simulink model "Katex_FullCar_R2017b_V03"  (R2026a)
settings: Solver=ode1  StopTime=1000  FixedStep=Ts  EnableMultiTasking=on
PostLoadFcn:
  | , if any(exist('dsrtsu_mdlpostloadfcn', 'file') == [2, 3, 6]), try dsrtsu_mdlpostloadfcn('Execute', bdroot); catch fprintf('Error in PostLoadFcn (dsrtsu_mdlpostloadfcn) for model "%s":\n %s\n', bdroot, lasterr); end, end,
  | , if any(exist('dsrtsu_mdlpostloadfcn', 'file') ~= 0), dsrtsu_mdlpostloadfcn('Execute', bdroot); end,
InitFcn:
  | , if any(exist('rtifpga_mdlclblib', 'file') ~= 0), rtifpga_mdlclblib('Init', bdroot); end,
  | 
  | 
  | init
undefined symbols (not defined in the file): locklim_sus, roundN, Ts
libraries: sl_discontinuities x29, simulink_extras x26, simulink x22, mjLib x1
(part 7 of 10)

== system Katex_FullCar_R2017b_V03/DGIST/_Low_Level_Ctrl/Suspension_Low_Level_Controller/Velocity Mode/Sus_LoadVel_2_MotorRPM/LPF2 ==
  note: LPF : tau = 1/(2*pi*fc)
  note: y(n) = [Ts*{x(n)+x(n-1)}+(2*tau-Ts)*y(n-1)]/(2*tau+Ts)
  note: H(s) = 1/(tau*s+1)
  note: s = 2/Ts*(z-1)/(z+1)
  In : Inport
  fc : Inport  Port=2
  Constant : Constant  Value=Ts  SampleTime=Ts
  Constant1 : Constant  SampleTime=Ts
  Product1 : Product  Inputs=*/  RndMeth=Zero
  Product11 : Product  RndMeth=Zero
  Product2 : Product  Inputs=*/  RndMeth=Zero
  Sum1 : Sum  Inputs=+-  InputSameDT=on  SaturateOnIntegerOverflow=on  OutDataTypeStr=Inherit: Same as first input
  Sum2 : Sum  InputSameDT=on  SaturateOnIntegerOverflow=on  OutDataTypeStr=Inherit: Same as first input
  Sum3 : Sum  InputSameDT=on  SaturateOnIntegerOverflow=on  OutDataTypeStr=Inherit: Same as first input
  Sum4 : Sum  InputSameDT=on  SaturateOnIntegerOverflow=on  OutDataTypeStr=Inherit: Same as first input
  d : UnitDelay  SampleTime=Ts
  d1 : UnitDelay  SampleTime=Ts
  gain : Gain  Gain=Ts  SaturateOnIntegerOverflow=on  OutDataTypeStr=Inherit: Same as input  ParamDataTypeStr=Inherit: Same as input
  gain1 : Gain  Gain=2  SaturateOnIntegerOverflow=on  OutDataTypeStr=Inherit: Same as input  ParamDataTypeStr=Inherit: Same as input
  gain2 : Gain  Gain=2*pi  SaturateOnIntegerOverflow=on  OutDataTypeStr=Inherit: Same as input  ParamDataTypeStr=Inherit: Same as input
  Out : Outport  VectorParamsAs1DForOutWhenUnconnected=off
  wires:
  In/1 -> Sum3/1, d1/1
  d1/1 -> Sum3/2
  Sum3/1 -> gain/1
  gain/1 -> Sum2/1
  Product11/1 -> Sum2/2
  Sum1/1 -> Product11/1
  Constant/1 -> Sum1/2, Sum4/2
  fc/1 -> gain2/1
  gain1/1 -> Sum1/1, Sum4/1
  d/1 -> Product11/2
  Sum2/1 -> Product1/1
  Sum4/1 -> Product1/2
  Product1/1 -> Out/1, d/1
  Product2/1 -> gain1/1
  Constant1/1 -> Product2/1
  gain2/1 -> Product2/2

== system Katex_FullCar_R2017b_V03/DGIST/_Low_Level_Ctrl/Suspension_Low_Level_Controller/Velocity Mode/Sus_LoadVel_2_MotorRPM1/LPF2 ==
  note: LPF : tau = 1/(2*pi*fc)
  note: y(n) = [Ts*{x(n)+x(n-1)}+(2*tau-Ts)*y(n-1)]/(2*tau+Ts)
  note: H(s) = 1/(tau*s+1)
  note: s = 2/Ts*(z-1)/(z+1)
  In : Inport
  fc : Inport  Port=2
  Constant : Constant  Value=Ts  SampleTime=Ts
  Constant1 : Constant  SampleTime=Ts
  Product1 : Product  Inputs=*/  RndMeth=Zero
  Product11 : Product  RndMeth=Zero
  Product2 : Product  Inputs=*/  RndMeth=Zero
  Sum1 : Sum  Inputs=+-  InputSameDT=on  SaturateOnIntegerOverflow=on  OutDataTypeStr=Inherit: Same as first input
  Sum2 : Sum  InputSameDT=on  SaturateOnIntegerOverflow=on  OutDataTypeStr=Inherit: Same as first input
  Sum3 : Sum  InputSameDT=on  SaturateOnIntegerOverflow=on  OutDataTypeStr=Inherit: Same as first input
  Sum4 : Sum  InputSameDT=on  SaturateOnIntegerOverflow=on  OutDataTypeStr=Inherit: Same as first input
  d : UnitDelay  SampleTime=Ts
  d1 : UnitDelay  SampleTime=Ts
  gain : Gain  Gain=Ts  SaturateOnIntegerOverflow=on  OutDataTypeStr=Inherit: Same as input  ParamDataTypeStr=Inherit: Same as input
  gain1 : Gain  Gain=2  SaturateOnIntegerOverflow=on  OutDataTypeStr=Inherit: Same as input  ParamDataTypeStr=Inherit: Same as input
  gain2 : Gain  Gain=2*pi  SaturateOnIntegerOverflow=on  OutDataTypeStr=Inherit: Same as input  ParamDataTypeStr=Inherit: Same as input
  Out : Outport  VectorParamsAs1DForOutWhenUnconnected=off
  wires:
  In/1 -> Sum3/1, d1/1
  d1/1 -> Sum3/2
  Sum3/1 -> gain/1
  gain/1 -> Sum2/1
  Product11/1 -> Sum2/2
  Sum1/1 -> Product11/1
  Constant/1 -> Sum1/2, Sum4/2
  fc/1 -> gain2/1
  gain1/1 -> Sum1/1, Sum4/1
  d/1 -> Product11/2
  Sum2/1 -> Product1/1
  Sum4/1 -> Product1/2
  Product1/1 -> Out/1, d/1
  Product2/1 -> gain1/1
  Constant1/1 -> Product2/1
  gain2/1 -> Product2/2

== system Katex_FullCar_R2017b_V03/DGIST/_Low_Level_Ctrl/Suspension_Low_Level_Controller/Velocity Mode/Sus_LoadVel_2_MotorRPM2/LPF2 ==
  note: LPF : tau = 1/(2*pi*fc)
  note: y(n) = [Ts*{x(n)+x(n-1)}+(2*tau-Ts)*y(n-1)]/(2*tau+Ts)
  note: H(s) = 1/(tau*s+1)
  note: s = 2/Ts*(z-1)/(z+1)
  In : Inport
  fc : Inport  Port=2
  Constant : Constant  Value=Ts  SampleTime=Ts
  Constant1 : Constant  SampleTime=Ts
  Product1 : Product  Inputs=*/  RndMeth=Zero
  Product11 : Product  RndMeth=Zero
  Product2 : Product  Inputs=*/  RndMeth=Zero
  Sum1 : Sum  Inputs=+-  InputSameDT=on  SaturateOnIntegerOverflow=on  OutDataTypeStr=Inherit: Same as first input
  Sum2 : Sum  InputSameDT=on  SaturateOnIntegerOverflow=on  OutDataTypeStr=Inherit: Same as first input
  Sum3 : Sum  InputSameDT=on  SaturateOnIntegerOverflow=on  OutDataTypeStr=Inherit: Same as first input
  Sum4 : Sum  InputSameDT=on  SaturateOnIntegerOverflow=on  OutDataTypeStr=Inherit: Same as first input
  d : UnitDelay  SampleTime=Ts
  d1 : UnitDelay  SampleTime=Ts
  gain : Gain  Gain=Ts  SaturateOnIntegerOverflow=on  OutDataTypeStr=Inherit: Same as input  ParamDataTypeStr=Inherit: Same as input
  gain1 : Gain  Gain=2  SaturateOnIntegerOverflow=on  OutDataTypeStr=Inherit: Same as input  ParamDataTypeStr=Inherit: Same as input
  gain2 : Gain  Gain=2*pi  SaturateOnIntegerOverflow=on  OutDataTypeStr=Inherit: Same as input  ParamDataTypeStr=Inherit: Same as input
  Out : Outport  VectorParamsAs1DForOutWhenUnconnected=off
  wires:
  In/1 -> Sum3/1, d1/1
  d1/1 -> Sum3/2
  Sum3/1 -> gain/1
  gain/1 -> Sum2/1
  Product11/1 -> Sum2/2
  Sum1/1 -> Product11/1
  Constant/1 -> Sum1/2, Sum4/2
  fc/1 -> gain2/1
  gain1/1 -> Sum1/1, Sum4/1
  d/1 -> Product11/2
  Sum2/1 -> Product1/1
  Sum4/1 -> Product1/2
  Product1/1 -> Out/1, d/1
  Product2/1 -> gain1/1
  Constant1/1 -> Product2/1
  gain2/1 -> Product2/2

== system Katex_FullCar_R2017b_V03/DGIST/_Low_Level_Ctrl/Suspension_Low_Level_Controller/Velocity Mode/Sus_LoadVel_2_MotorRPM3/LPF2 ==
  note: LPF : tau = 1/(2*pi*fc)
  note: y(n) = [Ts*{x(n)+x(n-1)}+(2*tau-Ts)*y(n-1)]/(2*tau+Ts)
  note: H(s) = 1/(tau*s+1)
  note: s = 2/Ts*(z-1)/(z+1)
  In : Inport
  fc : Inport  Port=2
  Constant : Constant  Value=Ts  SampleTime=Ts
  Constant1 : Constant  SampleTime=Ts
  Product1 : Product  Inputs=*/  RndMeth=Zero
  Product11 : Product  RndMeth=Zero
  Product2 : Product  Inputs=*/  RndMeth=Zero
  Sum1 : Sum  Inputs=+-  InputSameDT=on  SaturateOnIntegerOverflow=on  OutDataTypeStr=Inherit: Same as first input
  Sum2 : Sum  InputSameDT=on  SaturateOnIntegerOverflow=on  OutDataTypeStr=Inherit: Same as first input
  Sum3 : Sum  InputSameDT=on  SaturateOnIntegerOverflow=on  OutDataTypeStr=Inherit: Same as first input
  Sum4 : Sum  InputSameDT=on  SaturateOnIntegerOverflow=on  OutDataTypeStr=Inherit: Same as first input
  d : UnitDelay  SampleTime=Ts
  d1 : UnitDelay  SampleTime=Ts
  gain : Gain  Gain=Ts  SaturateOnIntegerOverflow=on  OutDataTypeStr=Inherit: Same as input  ParamDataTypeStr=Inherit: Same as input
  gain1 : Gain  Gain=2  SaturateOnIntegerOverflow=on  OutDataTypeStr=Inherit: Same as input  ParamDataTypeStr=Inherit: Same as input
  gain2 : Gain  Gain=2*pi  SaturateOnIntegerOverflow=on  OutDataTypeStr=Inherit: Same as input  ParamDataTypeStr=Inherit: Same as input
  Out : Outport  VectorParamsAs1DForOutWhenUnconnected=off
  wires:
  In/1 -> Sum3/1, d1/1
  d1/1 -> Sum3/2
  Sum3/1 -> gain/1
  gain/1 -> Sum2/1
  Product11/1 -> Sum2/2
  Sum1/1 -> Product11/1
  Constant/1 -> Sum1/2, Sum4/2
  fc/1 -> gain2/1
  gain1/1 -> Sum1/1, Sum4/1
  d/1 -> Product11/2
  Sum2/1 -> Product1/1
  Sum4/1 -> Product1/2
  Product1/1 -> Out/1, d/1
  Product2/1 -> gain1/1
  Constant1/1 -> Product2/1
  gain2/1 -> Product2/2

== system Katex_FullCar_R2017b_V03/MuJoCo Interface/FL_Motor_Control/Drv_Driver/Velocity Mode/FL_vel_velocity_motor_driver/poleplacement(PI)1 ==
  error : Inport
  zeta : Inport  Port=2
  freq : Inport  Port=3
  anti_windup : Inport  Port=4
  2*zeta*wn*J : Product  Inputs=3
  2*zeta*wn*J1 : Product
  2*zeta*wn*J2 : Product
  Add : Sum  Inputs=+-
  Add1 : Sum
  Constant3 : Constant  Value=0.05
  Constant4 : Constant  Value=0.9
  Display : Display
  Display1 : Display
  Gain : Gain  Gain=2
  Integ : Subsystem
  Product : Product  Inputs=*/
  Sum : Sum  Inputs=|+-
  Unit Delay : UnitDelay  SampleTime=-1
  wn : Gain  Gain=2*pi
  wn^2*J : Product  Inputs=3
  controlgain : Outport
  wires:
  Unit Delay/1 -> Sum/2
  [local_Kp] -> Product/2
  Product/1 -> Unit Delay/1
  anti_windup/1 -> Product/1
  Sum/1 -> Integ/1(error)
  2*zeta*wn*J1/1 -> Add1/2
  2*zeta*wn*J2/1 -> Add1/1
  Add1/1 -> controlgain/1
  [local_Kp] -> 2*zeta*wn*J2/1
  [local_Ki] -> 2*zeta*wn*J1/2
  Integ/1(Out1) -> 2*zeta*wn*J1/1
  error/1 -> 2*zeta*wn*J2/2, Sum/1
  wn^2*J/1 -> Display1/1, [local_Ki]
  [Local_J] -> wn^2*J/3
  Add/1 -> Display/1, [local_Kp]
  wn/1 -> wn^2*J/1, wn^2*J/2, 2*zeta*wn*J/3
  Gain/1 -> 2*zeta*wn*J/1
  zeta/1 -> Gain/1
  [Local_J] -> 2*zeta*wn*J/2
  2*zeta*wn*J/1 -> Add/1
  [Local_B] -> Add/2
  freq/1 -> wn/1
  Constant4/1 -> [Local_B]
  Constant3/1 -> [Local_J]

== system Katex_FullCar_R2017b_V03/MuJoCo Interface/FL_Motor_Control/Str_Driver/Position Mode/FL_str_position_motor_driver/poleplacement(PD)+I ==
  error : Inport
  zeta : Inport  Port=2
  freq : Inport  Port=3
  velocity_rad_s : Inport  Port=4
  2*zeta*wn*J : Product  Inputs=3
  2*zeta*wn*J1 : Product
  2*zeta*wn*J2 : Product
  Add : Sum  Inputs=+-
  Add1 : Sum
  Constant3 : Constant
  Constant4 : Constant  Value=10
  Display : Display
  Display1 : Display
  Gain : Gain  Gain=2
  Gain1 : Gain  Gain=-1
  Saturation5 : Saturate  UpperLimit=100  LowerLimit=-100
  wn : Gain  Gain=2*pi
  wn^2*J : Product  Inputs=3
  controlgain : Outport
  wires:
  2*zeta*wn*J1/1 -> Add1/2
  Saturation5/1 -> controlgain/1  "Usat"
  Add1/1 -> Saturation5/1
  Gain1/1 -> 2*zeta*wn*J1/2
  2*zeta*wn*J2/1 -> Add1/1
  [local_Kp] -> 2*zeta*wn*J2/1
  [local_Kd] -> Gain1/1
  error/1 -> 2*zeta*wn*J2/2
  wn^2*J/1 -> Display1/1, [local_Kp]
  [Local_J] -> wn^2*J/3
  Add/1 -> Display/1, [local_Kd]
  wn/1 -> wn^2*J/1, wn^2*J/2, 2*zeta*wn*J/3
  Gain/1 -> 2*zeta*wn*J/1
  zeta/1 -> Gain/1
  [Local_J] -> 2*zeta*wn*J/2
  2*zeta*wn*J/1 -> Add/1
  [Local_B] -> Add/2
  freq/1 -> wn/1
  Constant4/1 -> [Local_B]
  Constant3/1 -> [Local_J]
  velocity_rad_s/1 -> 2*zeta*wn*J1/1

== system Katex_FullCar_R2017b_V03/MuJoCo Interface/FL_Motor_Control/Sus_Driver/Position Mode/FL_sus_position_motor_driver/poleplacement(PD)+I ==
  error : Inport
  zeta : Inport  Port=2
  freq : Inport  Port=3
  velocity_rad_s : Inport  Port=4
  2*zeta*wn*J : Product  Inputs=3
  2*zeta*wn*J1 : Product
  2*zeta*wn*J2 : Product
  Add : Sum  Inputs=+-
  Add1 : Sum  Inputs=+++
  Add2 : Sum  Inputs=+-
  Constant : Constant
  Constant3 : Constant  Value=0.05
  Constant4 : Constant  Value=1.05
  Display : Display
  Display1 : Display
  Gain : Gain  Gain=2
  Gain1 : Gain  Gain=-1
  Integ : Subsystem
  Product : Product  Inputs=*/
  Saturation5 : Saturate  UpperLimit=100  LowerLimit=-100
  Sum : Sum  Inputs=|+-
  Unit Delay : UnitDelay  SampleTime=-1
  ki : Product
  wn : Gain  Gain=2*pi
  wn^2*J : Product  Inputs=3
  controlgain : Outport
  wires:
  Constant3/1 -> [Local_J]
  Constant4/1 -> [Local_B]
  freq/1 -> wn/1
  [Local_B] -> Add/2
  2*zeta*wn*J/1 -> Add/1
  [Local_J] -> 2*zeta*wn*J/2
  zeta/1 -> Gain/1
  Gain/1 -> 2*zeta*wn*J/1
  wn/1 -> 2*zeta*wn*J/3, wn^2*J/2, wn^2*J/1
  Add/1 -> [local_Kd], Display/1
  [Local_J] -> wn^2*J/3
  wn^2*J/1 -> [local_Kp], Display1/1
  error/1 -> 2*zeta*wn*J2/2, Sum/1
  [local_Kd] -> Gain1/1
  [local_Kp] -> 2*zeta*wn*J2/1
  2*zeta*wn*J2/1 -> Add1/1
  Gain1/1 -> 2*zeta*wn*J1/2
  2*zeta*wn*J1/1 -> Add1/3
  ki/1 -> Add1/2
  Constant/1 -> ki/2
  Integ/1(Out1) -> ki/1
  Add1/1 -> Add2/1, Saturation5/1
  Saturation5/1 -> Add2/2, controlgain/1  "Usat"
  Add2/1 -> Product/1
  [local_Kp] -> Product/2
  Sum/1 -> Integ/1(error)
  Product/1 -> Unit Delay/1
  Unit Delay/1 -> Sum/2
  velocity_rad_s/1 -> 2*zeta*wn*J1/1

== system Katex_FullCar_R2017b_V03/MuJoCo Interface/FR_Motor_Control/Drv_Driver/Velocity Mode/FR_vel_velocity_motor_driver/poleplacement(PI)1 ==
  error : Inport
  zeta : Inport  Port=2
  freq : Inport  Port=3
  anti_windup : Inport  Port=4
  2*zeta*wn*J : Product  Inputs=3
  2*zeta*wn*J1 : Product
  2*zeta*wn*J2 : Product
  Add : Sum  Inputs=+-
  Add1 : Sum
  Constant3 : Constant  Value=0.05
  Constant4 : Constant  Value=0.9
  Display : Display
  Display1 : Display
  Gain : Gain  Gain=2
  Integ : Subsystem
  Product : Product  Inputs=*/
  Sum : Sum  Inputs=|+-
  Unit Delay : UnitDelay  SampleTime=-1
  wn : Gain  Gain=2*pi
  wn^2*J : Product  Inputs=3
  controlgain : Outport
  wires:
  Constant3/1 -> [Local_J]
  Constant4/1 -> [Local_B]
  freq/1 -> wn/1
  [Local_B] -> Add/2
  2*zeta*wn*J/1 -> Add/1
  [Local_J] -> 2*zeta*wn*J/2
  zeta/1 -> Gain/1
  Gain/1 -> 2*zeta*wn*J/1
  wn/1 -> 2*zeta*wn*J/3, wn^2*J/2, wn^2*J/1
  Add/1 -> [local_Kp], Display/1
  [Local_J] -> wn^2*J/3
  wn^2*J/1 -> [local_Ki], Display1/1
  error/1 -> Sum/1, 2*zeta*wn*J2/2
  Integ/1(Out1) -> 2*zeta*wn*J1/1
  [local_Ki] -> 2*zeta*wn*J1/2
  [local_Kp] -> 2*zeta*wn*J2/1
  Add1/1 -> controlgain/1
  2*zeta*wn*J2/1 -> Add1/1
  2*zeta*wn*J1/1 -> Add1/2
  Sum/1 -> Integ/1(error)
  anti_windup/1 -> Product/1
  Product/1 -> Unit Delay/1
  [local_Kp] -> Product/2
  Unit Delay/1 -> Sum/2

== system Katex_FullCar_R2017b_V03/MuJoCo Interface/FR_Motor_Control/Str_Driver/Position Mode/FR_str_position_motor_driver/poleplacement(PD)+I ==
  error : Inport
  zeta : Inport  Port=2
  freq : Inport  Port=3
  velocity_rad_s : Inport  Port=4
  2*zeta*wn*J : Product  Inputs=3
  2*zeta*wn*J1 : Product
  2*zeta*wn*J2 : Product
  Add : Sum  Inputs=+-
  Add1 : Sum
  Constant3 : Constant
  Constant4 : Constant  Value=10
  Display : Display
  Display1 : Display
  Gain : Gain  Gain=2
  Gain1 : Gain  Gain=-1
  Saturation5 : Saturate  UpperLimit=100  LowerLimit=-100
  wn : Gain  Gain=2*pi
  wn^2*J : Product  Inputs=3
  controlgain : Outport
  wires:
  velocity_rad_s/1 -> 2*zeta*wn*J1/1
  Constant3/1 -> [Local_J]
  Constant4/1 -> [Local_B]
  freq/1 -> wn/1
  [Local_B] -> Add/2
  2*zeta*wn*J/1 -> Add/1
  [Local_J] -> 2*zeta*wn*J/2
  zeta/1 -> Gain/1
  Gain/1 -> 2*zeta*wn*J/1
  wn/1 -> 2*zeta*wn*J/3, wn^2*J/2, wn^2*J/1
  Add/1 -> [local_Kd], Display/1
  [Local_J] -> wn^2*J/3
  wn^2*J/1 -> [local_Kp], Display1/1
  error/1 -> 2*zeta*wn*J2/2
  [local_Kd] -> Gain1/1
  [local_Kp] -> 2*zeta*wn*J2/1
  2*zeta*wn*J2/1 -> Add1/1
  Gain1/1 -> 2*zeta*wn*J1/2
  Add1/1 -> Saturation5/1
  Saturation5/1 -> controlgain/1  "Usat"
  2*zeta*wn*J1/1 -> Add1/2

== system Katex_FullCar_R2017b_V03/MuJoCo Interface/FR_Motor_Control/Sus_Driver/Position Mode/FR_sus_position_motor_driver/poleplacement(PD)+I ==
  error : Inport
  zeta : Inport  Port=2
  freq : Inport  Port=3
  velocity_rad_s : Inport  Port=4
  2*zeta*wn*J : Product  Inputs=3
  2*zeta*wn*J1 : Product
  2*zeta*wn*J2 : Product
  Add : Sum  Inputs=+-
  Add1 : Sum  Inputs=+++
  Add2 : Sum  Inputs=+-
  Constant : Constant
  Constant3 : Constant  Value=0.05
  Constant4 : Constant  Value=1.05
  Display : Display
  Display1 : Display
  Gain : Gain  Gain=2
  Gain1 : Gain  Gain=-1
  Integ : Subsystem
  Product : Product  Inputs=*/
  Saturation5 : Saturate  UpperLimit=100  LowerLimit=-100
  Sum : Sum  Inputs=|+-
  Unit Delay : UnitDelay  SampleTime=-1
  ki : Product
  wn : Gain  Gain=2*pi
  wn^2*J : Product  Inputs=3
  controlgain : Outport
  wires:
  velocity_rad_s/1 -> 2*zeta*wn*J1/1
  Unit Delay/1 -> Sum/2
  Product/1 -> Unit Delay/1
  Sum/1 -> Integ/1(error)
  [local_Kp] -> Product/2
  Add2/1 -> Product/1
  Saturation5/1 -> controlgain/1, Add2/2  "Usat"
  Add1/1 -> Saturation5/1, Add2/1
  Integ/1(Out1) -> ki/1
  Constant/1 -> ki/2
  ki/1 -> Add1/2
  2*zeta*wn*J1/1 -> Add1/3
  Gain1/1 -> 2*zeta*wn*J1/2
  2*zeta*wn*J2/1 -> Add1/1
  [local_Kp] -> 2*zeta*wn*J2/1
  [local_Kd] -> Gain1/1
  error/1 -> Sum/1, 2*zeta*wn*J2/2
  wn^2*J/1 -> Display1/1, [local_Kp]
  [Local_J] -> wn^2*J/3
  Add/1 -> Display/1, [local_Kd]
  wn/1 -> wn^2*J/1, wn^2*J/2, 2*zeta*wn*J/3
  Gain/1 -> 2*zeta*wn*J/1
  zeta/1 -> Gain/1
  [Local_J] -> 2*zeta*wn*J/2
  2*zeta*wn*J/1 -> Add/1
  [Local_B] -> Add/2
  freq/1 -> wn/1
  Constant4/1 -> [Local_B]
  Constant3/1 -> [Local_J]

== system Katex_FullCar_R2017b_V03/MuJoCo Interface/RL_Motor_Control/Drv_Driver/Velocity Mode/RL_vel_velocity_motor_driver/poleplacement(PI)1 ==
  error : Inport
  zeta : Inport  Port=2
  freq : Inport  Port=3
  anti_windup : Inport  Port=4
  2*zeta*wn*J : Product  Inputs=3
  2*zeta*wn*J1 : Product
  2*zeta*wn*J2 : Product
  Add : Sum  Inputs=+-
  Add1 : Sum
  Constant3 : Constant  Value=0.05
  Constant4 : Constant  Value=0.9
  Display : Display
  Display1 : Display
  Gain : Gain  Gain=2
  Integ : Subsystem
  Product : Product  Inputs=*/
  Sum : Sum  Inputs=|+-
  Unit Delay : UnitDelay  SampleTime=-1
  wn : Gain  Gain=2*pi
  wn^2*J : Product  Inputs=3
  controlgain : Outport
  wires:
  Constant3/1 -> [Local_J]
  Constant4/1 -> [Local_B]
  freq/1 -> wn/1
  [Local_B] -> Add/2
  2*zeta*wn*J/1 -> Add/1
  [Local_J] -> 2*zeta*wn*J/2
  zeta/1 -> Gain/1
  Gain/1 -> 2*zeta*wn*J/1
  wn/1 -> 2*zeta*wn*J/3, wn^2*J/2, wn^2*J/1
  Add/1 -> [local_Kp], Display/1
  [Local_J] -> wn^2*J/3
  wn^2*J/1 -> [local_Ki], Display1/1
  error/1 -> Sum/1, 2*zeta*wn*J2/2
  Integ/1(Out1) -> 2*zeta*wn*J1/1
  [local_Ki] -> 2*zeta*wn*J1/2
  [local_Kp] -> 2*zeta*wn*J2/1
  Add1/1 -> controlgain/1
  2*zeta*wn*J2/1 -> Add1/1
  2*zeta*wn*J1/1 -> Add1/2
  Sum/1 -> Integ/1(error)
  anti_windup/1 -> Product/1
  Product/1 -> Unit Delay/1
  [local_Kp] -> Product/2
  Unit Delay/1 -> Sum/2

== system Katex_FullCar_R2017b_V03/MuJoCo Interface/RL_Motor_Control/Str_Driver/Position Mode/RL_str_position_motor_driver/poleplacement(PD)+I ==
  error : Inport
  zeta : Inport  Port=2
  freq : Inport  Port=3
  velocity_rad_s : Inport  Port=4
  2*zeta*wn*J : Product  Inputs=3
  2*zeta*wn*J1 : Product
  2*zeta*wn*J2 : Product
  Add : Sum  Inputs=+-
  Add1 : Sum
  Constant3 : Constant
  Constant4 : Constant  Value=10
  Display : Display
  Display1 : Display
  Gain : Gain  Gain=2
  Gain1 : Gain  Gain=-1
  Saturation5 : Saturate  UpperLimit=100  LowerLimit=-100
  wn : Gain  Gain=2*pi
  wn^2*J : Product  Inputs=3
  controlgain : Outport
  wires:
  velocity_rad_s/1 -> 2*zeta*wn*J1/1
  Constant3/1 -> [Local_J]
  Constant4/1 -> [Local_B]
  freq/1 -> wn/1
  [Local_B] -> Add/2
  2*zeta*wn*J/1 -> Add/1
  [Local_J] -> 2*zeta*wn*J/2
  zeta/1 -> Gain/1
  Gain/1 -> 2*zeta*wn*J/1
  wn/1 -> 2*zeta*wn*J/3, wn^2*J/2, wn^2*J/1
  Add/1 -> [local_Kd], Display/1
  [Local_J] -> wn^2*J/3
  wn^2*J/1 -> [local_Kp], Display1/1
  error/1 -> 2*zeta*wn*J2/2
  [local_Kd] -> Gain1/1
  [local_Kp] -> 2*zeta*wn*J2/1
  2*zeta*wn*J2/1 -> Add1/1
  Gain1/1 -> 2*zeta*wn*J1/2
  Add1/1 -> Saturation5/1
  Saturation5/1 -> controlgain/1  "Usat"
  2*zeta*wn*J1/1 -> Add1/2

== system Katex_FullCar_R2017b_V03/MuJoCo Interface/RL_Motor_Control/Sus_Driver/Position Mode/RL_sus_position_motor_driver/poleplacement(PD)+I ==
  error : Inport
  zeta : Inport  Port=2
  freq : Inport  Port=3
  velocity_rad_s : Inport  Port=4
  2*zeta*wn*J : Product  Inputs=3
  2*zeta*wn*J1 : Product
  2*zeta*wn*J2 : Product
  Add : Sum  Inputs=+-
  Add1 : Sum  Inputs=+++
  Add2 : Sum  Inputs=+-
  Constant : Constant
  Constant3 : Constant  Value=0.05
  Constant4 : Constant  Value=1.05
  Display : Display
  Display1 : Display
  Gain : Gain  Gain=2
  Gain1 : Gain  Gain=-1
  Integ : Subsystem
  Product : Product  Inputs=*/
  Saturation5 : Saturate  UpperLimit=100  LowerLimit=-100
  Sum : Sum  Inputs=|+-
  Unit Delay : UnitDelay  SampleTime=-1
  ki : Product
  wn : Gain  Gain=2*pi
  wn^2*J : Product  Inputs=3
  controlgain : Outport
  wires:
  velocity_rad_s/1 -> 2*zeta*wn*J1/1
  Unit Delay/1 -> Sum/2
  Product/1 -> Unit Delay/1
  Sum/1 -> Integ/1(error)
  [local_Kp] -> Product/2
  Add2/1 -> Product/1
  Saturation5/1 -> controlgain/1, Add2/2  "Usat"
  Add1/1 -> Saturation5/1, Add2/1
  Integ/1(Out1) -> ki/1
  Constant/1 -> ki/2
  ki/1 -> Add1/2
  2*zeta*wn*J1/1 -> Add1/3
  Gain1/1 -> 2*zeta*wn*J1/2
  2*zeta*wn*J2/1 -> Add1/1
  [local_Kp] -> 2*zeta*wn*J2/1
  [local_Kd] -> Gain1/1
  error/1 -> Sum/1, 2*zeta*wn*J2/2
  wn^2*J/1 -> Display1/1, [local_Kp]
  [Local_J] -> wn^2*J/3
  Add/1 -> Display/1, [local_Kd]
  wn/1 -> wn^2*J/1, wn^2*J/2, 2*zeta*wn*J/3
  Gain/1 -> 2*zeta*wn*J/1
  zeta/1 -> Gain/1
  [Local_J] -> 2*zeta*wn*J/2
  2*zeta*wn*J/1 -> Add/1
  [Local_B] -> Add/2
  freq/1 -> wn/1
  Constant4/1 -> [Local_B]
  Constant3/1 -> [Local_J]

== system Katex_FullCar_R2017b_V03/MuJoCo Interface/RR_Motor_Control/Drv_Driver/Velocity Mode/RR_vel_velocity_motor_driver/poleplacement(PI)1 ==
  error : Inport
  zeta : Inport  Port=2
  freq : Inport  Port=3
  anti_windup : Inport  Port=4
  2*zeta*wn*J : Product  Inputs=3
  2*zeta*wn*J1 : Product
  2*zeta*wn*J2 : Product
  Add : Sum  Inputs=+-
  Add1 : Sum
  Constant3 : Constant  Value=0.05
  Constant4 : Constant  Value=0.9
  Display : Display
  Display1 : Display
  Gain : Gain  Gain=2
  Integ : Subsystem
  Product : Product  Inputs=*/
  Sum : Sum  Inputs=|+-
  Unit Delay : UnitDelay  SampleTime=-1
  wn : Gain  Gain=2*pi
  wn^2*J : Product  Inputs=3
  controlgain : Outport
  wires:
  Constant3/1 -> [Local_J]
  Constant4/1 -> [Local_B]
  freq/1 -> wn/1
  [Local_B] -> Add/2
  2*zeta*wn*J/1 -> Add/1
  [Local_J] -> 2*zeta*wn*J/2
  zeta/1 -> Gain/1
  Gain/1 -> 2*zeta*wn*J/1
  wn/1 -> 2*zeta*wn*J/3, wn^2*J/2, wn^2*J/1
  Add/1 -> [local_Kp], Display/1
  [Local_J] -> wn^2*J/3
  wn^2*J/1 -> [local_Ki], Display1/1
  error/1 -> Sum/1, 2*zeta*wn*J2/2
  Integ/1(Out1) -> 2*zeta*wn*J1/1
  [local_Ki] -> 2*zeta*wn*J1/2
  [local_Kp] -> 2*zeta*wn*J2/1
  Add1/1 -> controlgain/1
  2*zeta*wn*J2/1 -> Add1/1
  2*zeta*wn*J1/1 -> Add1/2
  Sum/1 -> Integ/1(error)
  anti_windup/1 -> Product/1
  Product/1 -> Unit Delay/1
  [local_Kp] -> Product/2
  Unit Delay/1 -> Sum/2

== system Katex_FullCar_R2017b_V03/MuJoCo Interface/RR_Motor_Control/Str_Driver/Position Mode/RR_str_position_motor_driver/poleplacement(PD)+I ==
  error : Inport
  zeta : Inport  Port=2
  freq : Inport  Port=3
  velocity_rad_s : Inport  Port=4
  2*zeta*wn*J : Product  Inputs=3
  2*zeta*wn*J1 : Product
  2*zeta*wn*J2 : Product
  Add : Sum  Inputs=+-
  Add1 : Sum
  Constant3 : Constant
  Constant4 : Constant  Value=10
  Display : Display
  Display1 : Display
  Gain : Gain  Gain=2
  Gain1 : Gain  Gain=-1
  Saturation5 : Saturate  UpperLimit=100  LowerLimit=-100
  wn : Gain  Gain=2*pi
  wn^2*J : Product  Inputs=3
  controlgain : Outport
  wires:
  velocity_rad_s/1 -> 2*zeta*wn*J1/1
  Constant3/1 -> [Local_J]
  Constant4/1 -> [Local_B]
  freq/1 -> wn/1
  [Local_B] -> Add/2
  2*zeta*wn*J/1 -> Add/1
  [Local_J] -> 2*zeta*wn*J/2
  zeta/1 -> Gain/1
  Gain/1 -> 2*zeta*wn*J/1
  wn/1 -> 2*zeta*wn*J/3, wn^2*J/2, wn^2*J/1
  Add/1 -> [local_Kd], Display/1
  [Local_J] -> wn^2*J/3
  wn^2*J/1 -> [local_Kp], Display1/1
  error/1 -> 2*zeta*wn*J2/2
  [local_Kd] -> Gain1/1
  [local_Kp] -> 2*zeta*wn*J2/1
  2*zeta*wn*J2/1 -> Add1/1
  Gain1/1 -> 2*zeta*wn*J1/2
  Add1/1 -> Saturation5/1
  Saturation5/1 -> controlgain/1  "Usat"
  2*zeta*wn*J1/1 -> Add1/2

== system Katex_FullCar_R2017b_V03/MuJoCo Interface/RR_Motor_Control/Sus_Driver/Position Mode/RR_sus_position_motor_driver/poleplacement(PD)+I ==
  error : Inport
  zeta : Inport  Port=2
  freq : Inport  Port=3
  velocity_rad_s : Inport  Port=4
  2*zeta*wn*J : Product  Inputs=3
  2*zeta*wn*J1 : Product
  2*zeta*wn*J2 : Product
  Add : Sum  Inputs=+-
  Add1 : Sum  Inputs=+++
  Add2 : Sum  Inputs=+-
  Constant : Constant
  Constant3 : Constant  Value=0.05
  Constant4 : Constant  Value=1.05
  Display : Display
  Display1 : Display
  Gain : Gain  Gain=2
  Gain1 : Gain  Gain=-1
  Integ : Subsystem
  Product : Product  Inputs=*/
  Saturation5 : Saturate  UpperLimit=100  LowerLimit=-100
  Sum : Sum  Inputs=|+-
  Unit Delay : UnitDelay  SampleTime=-1
  ki : Product
  wn : Gain  Gain=2*pi
  wn^2*J : Product  Inputs=3
  controlgain : Outport
  wires:
  velocity_rad_s/1 -> 2*zeta*wn*J1/1
  Unit Delay/1 -> Sum/2
  Product/1 -> Unit Delay/1
  Sum/1 -> Integ/1(error)
  [local_Kp] -> Product/2
  Add2/1 -> Product/1
  Saturation5/1 -> controlgain/1, Add2/2  "Usat"
  Add1/1 -> Saturation5/1, Add2/1
  Integ/1(Out1) -> ki/1
  Constant/1 -> ki/2
  ki/1 -> Add1/2
  2*zeta*wn*J1/1 -> Add1/3
  Gain1/1 -> 2*zeta*wn*J1/2
  2*zeta*wn*J2/1 -> Add1/1
  [local_Kp] -> 2*zeta*wn*J2/1
  [local_Kd] -> Gain1/1
  error/1 -> Sum/1, 2*zeta*wn*J2/2
  wn^2*J/1 -> [local_Kp], Display1/1
  [Local_J] -> wn^2*J/3
  Add/1 -> Display/1, [local_Kd]
  wn/1 -> wn^2*J/1, wn^2*J/2, 2*zeta*wn*J/3
  Gain/1 -> 2*zeta*wn*J/1
  zeta/1 -> Gain/1
  [Local_J] -> 2*zeta*wn*J/2
  2*zeta*wn*J/1 -> Add/1
  [Local_B] -> Add/2
  freq/1 -> wn/1
  Constant4/1 -> [Local_B]
  Constant3/1 -> [Local_J]

== system Katex_FullCar_R2017b_V03/DGIST/_High_Level_Ctrl/Chassis_FB_ctrl/Slip contro FLl/Subsystem/Subsystem1/If Action Subsystem ==
  In1 : Inport
  Action Port : ActionPort  ActionPortLabel=if(u1 >= 0)
  Out1 : Outport  VectorParamsAs1DForOutWhenUnconnected=off
  wires:
  In1/1 -> Out1/1

== system Katex_FullCar_R2017b_V03/DGIST/_High_Level_Ctrl/Chassis_FB_ctrl/Slip contro FLl/Subsystem/Subsystem1/If Action Subsystem1 ==
  In1 : Inport
  Action Port : ActionPort  ActionPortLabel=elseif(u1<0)
  Out1 : Outport  VectorParamsAs1DForOutWhenUnconnected=off
  wires:
  In1/1 -> Out1/1

== system Katex_FullCar_R2017b_V03/DGIST/_High_Level_Ctrl/Chassis_FB_ctrl/Slip control FR/Subsystem/Subsystem1/If Action Subsystem ==
  In1 : Inport
  Action Port : ActionPort  ActionPortLabel=if(u1 >= 0)
  Out1 : Outport  VectorParamsAs1DForOutWhenUnconnected=off
  wires:
  In1/1 -> Out1/1

== system Katex_FullCar_R2017b_V03/DGIST/_High_Level_Ctrl/Chassis_FB_ctrl/Slip control FR/Subsystem/Subsystem1/If Action Subsystem1 ==
  In1 : Inport
  Action Port : ActionPort  ActionPortLabel=elseif(u1<0)
  Out1 : Outport  VectorParamsAs1DForOutWhenUnconnected=off
  wires:
  In1/1 -> Out1/1

== system Katex_FullCar_R2017b_V03/DGIST/_Low_Level_Ctrl/Driving_Low_Level_Controller/Torque Mode/Driving Wheel Control/DOB(omega)/Dot2 ==
  note: Dot
  in : Inport
  Sum1 : Sum  Inputs=+-  InputSameDT=on  SaturateOnIntegerOverflow=on  OutDataTypeStr=Inherit: Same as first input
  Sum2 : Sum  Inputs=+-  InputSameDT=on  SaturateOnIntegerOverflow=on  OutDataTypeStr=Inherit: Same as first input
  d : UnitDelay  SampleTime=Ts
  d1 : UnitDelay  SampleTime=Ts
  gain : Gain  Gain=2/Ts  SaturateOnIntegerOverflow=on  OutDataTypeStr=Inherit: Same as input  ParamDataTypeStr=Inherit: Same as input
  out : Outport  VectorParamsAs1DForOutWhenUnconnected=off
  wires:
  Sum1/1 -> d1/1, out/1
  d1/1 -> Sum1/2
  Sum2/1 -> gain/1
  in/1 -> d/1, Sum2/1
  d/1 -> Sum2/2
  gain/1 -> Sum1/1

== system Katex_FullCar_R2017b_V03/DGIST/_Low_Level_Ctrl/Driving_Low_Level_Controller/Torque Mode/Driving Wheel Control/DOB(omega)/LPF ==
  note: LPF : tau = 1/(2*pi*fc)
  note: y(n) = [Ts*{x(n)+x(n-1)}+(2*tau-Ts)*y(n-1)]/(2*tau+Ts)
  note: H(s) = 1/(tau*s+1)
  note: s = 2/Ts*(z-1)/(z+1)
  In : Inport
  fc : Inport  Port=2
  Constant : Constant  Value=Ts  SampleTime=Ts
  Constant1 : Constant  SampleTime=Ts
  Product1 : Product  Inputs=*/  RndMeth=Zero
  Product11 : Product  RndMeth=Zero
  Product2 : Product  Inputs=*/  RndMeth=Zero
  Sum1 : Sum  Inputs=+-  InputSameDT=on  SaturateOnIntegerOverflow=on  OutDataTypeStr=Inherit: Same as first input
  Sum2 : Sum  InputSameDT=on  SaturateOnIntegerOverflow=on  OutDataTypeStr=Inherit: Same as first input
  Sum3 : Sum  InputSameDT=on  SaturateOnIntegerOverflow=on  OutDataTypeStr=Inherit: Same as first input
  Sum4 : Sum  InputSameDT=on  SaturateOnIntegerOverflow=on  OutDataTypeStr=Inherit: Same as first input
  d : UnitDelay  SampleTime=Ts
  d1 : UnitDelay  SampleTime=Ts
  gain : Gain  Gain=Ts  SaturateOnIntegerOverflow=on  OutDataTypeStr=Inherit: Same as input  ParamDataTypeStr=Inherit: Same as input
  gain1 : Gain  Gain=2  SaturateOnIntegerOverflow=on  OutDataTypeStr=Inherit: Same as input  ParamDataTypeStr=Inherit: Same as input
  gain2 : Gain  Gain=2*pi  SaturateOnIntegerOverflow=on  OutDataTypeStr=Inherit: Same as input  ParamDataTypeStr=Inherit: Same as input
  Out : Outport  VectorParamsAs1DForOutWhenUnconnected=off
  wires:
  In/1 -> Sum3/1, d1/1
  d1/1 -> Sum3/2
  Sum3/1 -> gain/1
  gain/1 -> Sum2/1
  Product11/1 -> Sum2/2
  Sum1/1 -> Product11/1
  Constant/1 -> Sum1/2, Sum4/2
  fc/1 -> gain2/1
  gain1/1 -> Sum1/1, Sum4/1
  d/1 -> Product11/2
  Sum2/1 -> Product1/1
  Sum4/1 -> Product1/2
  Product1/1 -> Out/1, d/1
  Product2/1 -> gain1/1
  Constant1/1 -> Product2/1
  gain2/1 -> Product2/2

== system Katex_FullCar_R2017b_V03/DGIST/_Low_Level_Ctrl/Driving_Low_Level_Controller/Torque Mode/Driving Wheel Control/Feedforward(omega)/Dot2 ==
  note: Dot
  in : Inport
  Sum1 : Sum  Inputs=+-  InputSameDT=on  SaturateOnIntegerOverflow=on  OutDataTypeStr=Inherit: Same as first input
  Sum2 : Sum  Inputs=+-  InputSameDT=on  SaturateOnIntegerOverflow=on  OutDataTypeStr=Inherit: Same as first input
  d : UnitDelay  SampleTime=Ts
  d1 : UnitDelay  SampleTime=Ts
  gain : Gain  Gain=2/Ts  SaturateOnIntegerOverflow=on  OutDataTypeStr=Inherit: Same as input  ParamDataTypeStr=Inherit: Same as input
  out : Outport  VectorParamsAs1DForOutWhenUnconnected=off
  wires:
  Sum1/1 -> d1/1, out/1
  d1/1 -> Sum1/2
  Sum2/1 -> gain/1
  in/1 -> d/1, Sum2/1
  d/1 -> Sum2/2
  gain/1 -> Sum1/1

== system Katex_FullCar_R2017b_V03/DGIST/_Low_Level_Ctrl/Driving_Low_Level_Controller/Torque Mode/Driving Wheel Control/Feedforward(omega)/LPF ==
  note: LPF : tau = 1/(2*pi*fc)
  note: y(n) = [Ts*{x(n)+x(n-1)}+(2*tau-Ts)*y(n-1)]/(2*tau+Ts)
  note: H(s) = 1/(tau*s+1)
  note: s = 2/Ts*(z-1)/(z+1)
  In : Inport
  fc : Inport  Port=2
  Constant : Constant  Value=Ts  SampleTime=Ts
  Constant1 : Constant  SampleTime=Ts
  Product1 : Product  Inputs=*/  RndMeth=Zero
  Product11 : Product  RndMeth=Zero
  Product2 : Product  Inputs=*/  RndMeth=Zero
  Sum1 : Sum  Inputs=+-  InputSameDT=on  SaturateOnIntegerOverflow=on  OutDataTypeStr=Inherit: Same as first input
  Sum2 : Sum  InputSameDT=on  SaturateOnIntegerOverflow=on  OutDataTypeStr=Inherit: Same as first input
  Sum3 : Sum  InputSameDT=on  SaturateOnIntegerOverflow=on  OutDataTypeStr=Inherit: Same as first input
  Sum4 : Sum  InputSameDT=on  SaturateOnIntegerOverflow=on  OutDataTypeStr=Inherit: Same as first input
  d : UnitDelay  SampleTime=Ts
  d1 : UnitDelay  SampleTime=Ts
  gain : Gain  Gain=Ts  SaturateOnIntegerOverflow=on  OutDataTypeStr=Inherit: Same as input  ParamDataTypeStr=Inherit: Same as input
  gain1 : Gain  Gain=2  SaturateOnIntegerOverflow=on  OutDataTypeStr=Inherit: Same as input  ParamDataTypeStr=Inherit: Same as input
  gain2 : Gain  Gain=2*pi  SaturateOnIntegerOverflow=on  OutDataTypeStr=Inherit: Same as input  ParamDataTypeStr=Inherit: Same as input
  Out : Outport  VectorParamsAs1DForOutWhenUnconnected=off
  wires:
  In/1 -> Sum3/1, d1/1
  d1/1 -> Sum3/2
  Sum3/1 -> gain/1
  gain/1 -> Sum2/1
  Product11/1 -> Sum2/2
  Sum1/1 -> Product11/1
  Constant/1 -> Sum1/2, Sum4/2
  fc/1 -> gain2/1
  gain1/1 -> Sum1/1, Sum4/1
  d/1 -> Product11/2
  Sum2/1 -> Product1/1
  Sum4/1 -> Product1/2
  Product1/1 -> Out/1, d/1
  Product2/1 -> gain1/1
  Constant1/1 -> Product2/1
  gain2/1 -> Product2/2

== system Katex_FullCar_R2017b_V03/DGIST/_Low_Level_Ctrl/Driving_Low_Level_Controller/Torque Mode/Driving Wheel Control/Poleplacement(PI)1/Integrator1 ==
  note: Integrator
  in : Inport
  "Off : 0 On : 1" : Inport  Port=2
  Divide : Product  Inputs=**
  Sum1 : Sum  InputSameDT=on  SaturateOnIntegerOverflow=on  OutDataTypeStr=Inherit: Same as first input
  Sum2 : Sum  InputSameDT=on  SaturateOnIntegerOverflow=on  OutDataTypeStr=Inherit: Same as first input
  d : UnitDelay  SampleTime=Ts
  d1 : UnitDelay  SampleTime=Ts
  gain : Gain  Gain=Ts/2  SaturateOnIntegerOverflow=on  OutDataTypeStr=Inherit: Same as input  ParamDataTypeStr=Inherit: Same as input
  out : Outport  VectorParamsAs1DForOutWhenUnconnected=off
  wires:
  gain/1 -> Sum2/1
  Sum1/1 -> gain/1
  d1/1 -> Sum1/2
  in/1 -> d1/1, Sum1/1
  Sum2/1 -> Divide/1, out/1
  d/1 -> Sum2/2
  Divide/1 -> d/1
  "Off : 0 On : 1"/1 -> Divide/2

== system Katex_FullCar_R2017b_V03/DGIST/_Low_Level_Ctrl/Steering_Low_Level_Controller/Torque Mode/Steering Motor Control/DOB(omega)/Dot2 ==
  note: Dot
  in : Inport
  Sum1 : Sum  Inputs=+-  InputSameDT=on  SaturateOnIntegerOverflow=on  OutDataTypeStr=Inherit: Same as first input
  Sum2 : Sum  Inputs=+-  InputSameDT=on  SaturateOnIntegerOverflow=on  OutDataTypeStr=Inherit: Same as first input
  d : UnitDelay  SampleTime=Ts
  d1 : UnitDelay  SampleTime=Ts
  gain : Gain  Gain=2/Ts  SaturateOnIntegerOverflow=on  OutDataTypeStr=Inherit: Same as input  ParamDataTypeStr=Inherit: Same as input
  out : Outport  VectorParamsAs1DForOutWhenUnconnected=off
  wires:
  Sum1/1 -> d1/1, out/1
  d1/1 -> Sum1/2
  Sum2/1 -> gain/1
  in/1 -> d/1, Sum2/1
  d/1 -> Sum2/2
  gain/1 -> Sum1/1

== system Katex_FullCar_R2017b_V03/DGIST/_Low_Level_Ctrl/Steering_Low_Level_Controller/Torque Mode/Steering Motor Control/DOB(omega)/LPF ==
  note: LPF : tau = 1/(2*pi*fc)
  note: y(n) = [Ts*{x(n)+x(n-1)}+(2*tau-Ts)*y(n-1)]/(2*tau+Ts)
  note: H(s) = 1/(tau*s+1)
  note: s = 2/Ts*(z-1)/(z+1)
  In : Inport
  fc : Inport  Port=2
  Constant : Constant  Value=Ts  SampleTime=Ts
  Constant1 : Constant  SampleTime=Ts
  Product1 : Product  Inputs=*/  RndMeth=Zero
  Product11 : Product  RndMeth=Zero
  Product2 : Product  Inputs=*/  RndMeth=Zero
  Sum1 : Sum  Inputs=+-  InputSameDT=on  SaturateOnIntegerOverflow=on  OutDataTypeStr=Inherit: Same as first input
  Sum2 : Sum  InputSameDT=on  SaturateOnIntegerOverflow=on  OutDataTypeStr=Inherit: Same as first input
  Sum3 : Sum  InputSameDT=on  SaturateOnIntegerOverflow=on  OutDataTypeStr=Inherit: Same as first input
  Sum4 : Sum  InputSameDT=on  SaturateOnIntegerOverflow=on  OutDataTypeStr=Inherit: Same as first input
  d : UnitDelay  SampleTime=Ts
  d1 : UnitDelay  SampleTime=Ts
  gain : Gain  Gain=Ts  SaturateOnIntegerOverflow=on  OutDataTypeStr=Inherit: Same as input  ParamDataTypeStr=Inherit: Same as input
  gain1 : Gain  Gain=2  SaturateOnIntegerOverflow=on  OutDataTypeStr=Inherit: Same as input  ParamDataTypeStr=Inherit: Same as input
  gain2 : Gain  Gain=2*pi  SaturateOnIntegerOverflow=on  OutDataTypeStr=Inherit: Same as input  ParamDataTypeStr=Inherit: Same as input
  Out : Outport  VectorParamsAs1DForOutWhenUnconnected=off
  wires:
  In/1 -> Sum3/1, d1/1
  d1/1 -> Sum3/2
  Sum3/1 -> gain/1
  gain/1 -> Sum2/1
  Product11/1 -> Sum2/2
  Sum1/1 -> Product11/1
  Constant/1 -> Sum1/2, Sum4/2
  fc/1 -> gain2/1
  gain1/1 -> Sum1/1, Sum4/1
  d/1 -> Product11/2
  Sum2/1 -> Product1/1
  Sum4/1 -> Product1/2
  Product1/1 -> Out/1, d/1
  Product2/1 -> gain1/1
  Constant1/1 -> Product2/1
  gain2/1 -> Product2/2

== system Katex_FullCar_R2017b_V03/DGIST/_Low_Level_Ctrl/Steering_Low_Level_Controller/Torque Mode/Steering Motor Control/DOB(theta)/Dot ==
  note: Dot
  in : Inport
  Sum1 : Sum  Inputs=+-  InputSameDT=on  SaturateOnIntegerOverflow=on  OutDataTypeStr=Inherit: Same as first input
  Sum2 : Sum  Inputs=+-  InputSameDT=on  SaturateOnIntegerOverflow=on  OutDataTypeStr=Inherit: Same as first input
  d : UnitDelay  SampleTime=Ts
  d1 : UnitDelay  SampleTime=Ts
  gain : Gain  Gain=2/Ts  SaturateOnIntegerOverflow=on  OutDataTypeStr=Inherit: Same as input  ParamDataTypeStr=Inherit: Same as input
  out : Outport  VectorParamsAs1DForOutWhenUnconnected=off
  wires:
  Sum1/1 -> d1/1, out/1
  d1/1 -> Sum1/2
  Sum2/1 -> gain/1
  in/1 -> d/1, Sum2/1
  d/1 -> Sum2/2
  gain/1 -> Sum1/1

== system Katex_FullCar_R2017b_V03/DGIST/_Low_Level_Ctrl/Steering_Low_Level_Controller/Torque Mode/Steering Motor Control/DOB(theta)/Dot1 ==
  note: Dot
  in : Inport
  Sum1 : Sum  Inputs=+-  InputSameDT=on  SaturateOnIntegerOverflow=on  OutDataTypeStr=Inherit: Same as first input
  Sum2 : Sum  Inputs=+-  InputSameDT=on  SaturateOnIntegerOverflow=on  OutDataTypeStr=Inherit: Same as first input
  d : UnitDelay  SampleTime=Ts
  d1 : UnitDelay  SampleTime=Ts
  gain : Gain  Gain=2/Ts  SaturateOnIntegerOverflow=on  OutDataTypeStr=Inherit: Same as input  ParamDataTypeStr=Inherit: Same as input
  out : Outport  VectorParamsAs1DForOutWhenUnconnected=off
  wires:
  Sum1/1 -> d1/1, out/1
  d1/1 -> Sum1/2
  Sum2/1 -> gain/1
  in/1 -> d/1, Sum2/1
  d/1 -> Sum2/2
  gain/1 -> Sum1/1

== system Katex_FullCar_R2017b_V03/DGIST/_Low_Level_Ctrl/Steering_Low_Level_Controller/Torque Mode/Steering Motor Control/DOB(theta)/Dot2 ==
  note: Dot
  in : Inport
  Sum1 : Sum  Inputs=+-  InputSameDT=on  SaturateOnIntegerOverflow=on  OutDataTypeStr=Inherit: Same as first input
  Sum2 : Sum  Inputs=+-  InputSameDT=on  SaturateOnIntegerOverflow=on  OutDataTypeStr=Inherit: Same as first input
  d : UnitDelay  SampleTime=Ts
  d1 : UnitDelay  SampleTime=Ts
  gain : Gain  Gain=2/Ts  SaturateOnIntegerOverflow=on  OutDataTypeStr=Inherit: Same as input  ParamDataTypeStr=Inherit: Same as input
  out : Outport  VectorParamsAs1DForOutWhenUnconnected=off
  wires:
  Sum1/1 -> d1/1, out/1
  d1/1 -> Sum1/2
  Sum2/1 -> gain/1
  in/1 -> d/1, Sum2/1
  d/1 -> Sum2/2
  gain/1 -> Sum1/1

== system Katex_FullCar_R2017b_V03/DGIST/_Low_Level_Ctrl/Steering_Low_Level_Controller/Torque Mode/Steering Motor Control/DOB(theta)/Second order LPF ==
  note: y(n) = [Ts^2*w^2*{x(n)+2*x(n-1)+x(n-2)}-(2*w^2*Ts^2-8)*y(n-1)-(4+w^2*Ts^2+2*zeta*Ts*w)*y(n-2)]
      | /(4+w^2*Ts^2+2*zeta*Ts*w)
  note: H(s) = w^2/(s^2+2*zeta*w*s+w^2)
  note: s = 2/Ts*(z-1)/(z+1)
  In : Inport
  fc : Inport  Port=2
  zeta : Inport  Port=3
  Constant : Constant  Value=Ts  SampleTime=Ts
  Constant1 : Constant  Value=8  SampleTime=Ts
  Constant2 : Constant  Value=4  SampleTime=Ts
  Delay : Delay  InitialCondition=0  SampleTime=Ts
  Delay1 : Delay  DelayLength=1  InitialCondition=0  SampleTime=Ts
  Delay2 : Delay  DelayLength=1  InitialCondition=0  SampleTime=Ts
  Delay3 : Delay  InitialCondition=0  SampleTime=Ts
  Product1 : Product  Inputs=*/  RndMeth=Zero
  Product2 : Product  Inputs=4  RndMeth=Zero
  Product3 : Product  RndMeth=Zero
  Product4 : Product  RndMeth=Zero
  Sum1 : Sum  Inputs=+-  InputSameDT=on  SaturateOnIntegerOverflow=on  OutDataTypeStr=Inherit: Same as first input
  Sum2 : Sum  Inputs=+-  InputSameDT=on  SaturateOnIntegerOverflow=on  OutDataTypeStr=Inherit: Same as first input
  Sum3 : Sum  Inputs=+++  InputSameDT=on  SaturateOnIntegerOverflow=on  OutDataTypeStr=Inherit: Same as first input
  Sum4 : Sum  Inputs=+-  InputSameDT=on  SaturateOnIntegerOverflow=on  OutDataTypeStr=Inherit: Same as first input
  Sum5 : Sum  Inputs=+-+  InputSameDT=on  SaturateOnIntegerOverflow=on  OutDataTypeStr=Inherit: Same as first input
  Sum6 : Sum  Inputs=+++  InputSameDT=on  SaturateOnIntegerOverflow=on  OutDataTypeStr=Inherit: Same as first input
  gain1 : Gain  Gain=2  SaturateOnIntegerOverflow=on  OutDataTypeStr=Inherit: Same as input  ParamDataTypeStr=Inherit: Same as input
  gain2 : Gain  Gain=2*pi  SaturateOnIntegerOverflow=on  OutDataTypeStr=Inherit: Same as input  ParamDataTypeStr=Inherit: Same as input
  gain3 : Gain  Gain=2  SaturateOnIntegerOverflow=on  OutDataTypeStr=Inherit: Same as input  ParamDataTypeStr=Inherit: Same as input
  gain4 : Gain  Gain=4  SaturateOnIntegerOverflow=on  OutDataTypeStr=Inherit: Same as input  ParamDataTypeStr=Inherit: Same as input
  "x(n), x(n-1), x(n-2)" : Product  RndMeth=Zero
  y(n-1) : Product  RndMeth=Zero
  y(n-2) : Product  RndMeth=Zero
  Dist_hat : Outport  VectorParamsAs1DForOutWhenUnconnected=off
  wires:
  Product1/1 -> Dist_hat/1, Delay3/1, Delay2/1
  Sum2/1 -> Product1/1
  fc/1 -> gain2/1
  In/1 -> Delay1/1, Delay/1, Sum3/1
  gain2/1 -> Product3/1, Product2/2, Product2/1
  Constant/1 -> Product3/2, Product2/4, Product2/3
  Delay1/1 -> gain1/1
  gain1/1 -> Sum3/2
  Delay/1 -> Sum3/3
  Sum3/1 -> "x(n), x(n-1), x(n-2)"/1
  Product2/1 -> Sum5/1, Sum6/1, "x(n), x(n-1), x(n-2)"/2, gain3/1
  "x(n), x(n-1), x(n-2)"/1 -> Sum1/1
  Sum1/1 -> Sum2/1
  y(n-1)/1 -> Sum1/2
  Sum4/1 -> y(n-1)/1
  gain3/1 -> Sum4/1
  Constant1/1 -> Sum4/2
  Delay2/1 -> y(n-1)/2
  Product3/1 -> gain4/1
  Constant2/1 -> Sum5/3, Sum6/3
  Sum5/1 -> y(n-2)/1
  Delay3/1 -> y(n-2)/2
  y(n-2)/1 -> Sum2/2
  Sum6/1 -> Product1/2
  zeta/1 -> Product4/2
  gain4/1 -> Product4/1
  Product4/1 -> Sum6/2, Sum5/2

== system Katex_FullCar_R2017b_V03/DGIST/_Low_Level_Ctrl/Steering_Low_Level_Controller/Torque Mode/Steering Motor Control/Feedforward(omega)/Dot2 ==
  note: Dot
  in : Inport
  Sum1 : Sum  Inputs=+-  InputSameDT=on  SaturateOnIntegerOverflow=on  OutDataTypeStr=Inherit: Same as first input
  Sum2 : Sum  Inputs=+-  InputSameDT=on  SaturateOnIntegerOverflow=on  OutDataTypeStr=Inherit: Same as first input
  d : UnitDelay  SampleTime=Ts
  d1 : UnitDelay  SampleTime=Ts
  gain : Gain  Gain=2/Ts  SaturateOnIntegerOverflow=on  OutDataTypeStr=Inherit: Same as input  ParamDataTypeStr=Inherit: Same as input
  out : Outport  VectorParamsAs1DForOutWhenUnconnected=off
  wires:
  Sum1/1 -> d1/1, out/1
  d1/1 -> Sum1/2
  Sum2/1 -> gain/1
  in/1 -> d/1, Sum2/1
  d/1 -> Sum2/2
  gain/1 -> Sum1/1

== system Katex_FullCar_R2017b_V03/DGIST/_Low_Level_Ctrl/Steering_Low_Level_Controller/Torque Mode/Steering Motor Control/Feedforward(omega)/LPF ==
  note: LPF : tau = 1/(2*pi*fc)
  note: y(n) = [Ts*{x(n)+x(n-1)}+(2*tau-Ts)*y(n-1)]/(2*tau+Ts)
  note: H(s) = 1/(tau*s+1)
  note: s = 2/Ts*(z-1)/(z+1)
  In : Inport
  fc : Inport  Port=2
  Constant : Constant  Value=Ts  SampleTime=Ts
  Constant1 : Constant  SampleTime=Ts
  Product1 : Product  Inputs=*/  RndMeth=Zero
  Product11 : Product  RndMeth=Zero
  Product2 : Product  Inputs=*/  RndMeth=Zero
  Sum1 : Sum  Inputs=+-  InputSameDT=on  SaturateOnIntegerOverflow=on  OutDataTypeStr=Inherit: Same as first input
  Sum2 : Sum  InputSameDT=on  SaturateOnIntegerOverflow=on  OutDataTypeStr=Inherit: Same as first input
  Sum3 : Sum  InputSameDT=on  SaturateOnIntegerOverflow=on  OutDataTypeStr=Inherit: Same as first input
  Sum4 : Sum  InputSameDT=on  SaturateOnIntegerOverflow=on  OutDataTypeStr=Inherit: Same as first input
  d : UnitDelay  SampleTime=Ts
  d1 : UnitDelay  SampleTime=Ts
  gain : Gain  Gain=Ts  SaturateOnIntegerOverflow=on  OutDataTypeStr=Inherit: Same as input  ParamDataTypeStr=Inherit: Same as input
  gain1 : Gain  Gain=2  SaturateOnIntegerOverflow=on  OutDataTypeStr=Inherit: Same as input  ParamDataTypeStr=Inherit: Same as input
  gain2 : Gain  Gain=2*pi  SaturateOnIntegerOverflow=on  OutDataTypeStr=Inherit: Same as input  ParamDataTypeStr=Inherit: Same as input
  Out : Outport  VectorParamsAs1DForOutWhenUnconnected=off
  wires:
  In/1 -> Sum3/1, d1/1
  d1/1 -> Sum3/2
  Sum3/1 -> gain/1
  gain/1 -> Sum2/1
  Product11/1 -> Sum2/2
  Sum1/1 -> Product11/1
  Constant/1 -> Sum1/2, Sum4/2
  fc/1 -> gain2/1
  gain1/1 -> Sum1/1, Sum4/1
  d/1 -> Product11/2
  Sum2/1 -> Product1/1
  Sum4/1 -> Product1/2
  Product1/1 -> Out/1, d/1
  Product2/1 -> gain1/1
  Constant1/1 -> Product2/1
  gain2/1 -> Product2/2

== system Katex_FullCar_R2017b_V03/DGIST/_Low_Level_Ctrl/Steering_Low_Level_Controller/Torque Mode/Steering Motor Control/Feedforward(theta)/Dot ==
  note: Dot
  in : Inport
  Sum1 : Sum  Inputs=+-  InputSameDT=on  SaturateOnIntegerOverflow=on  OutDataTypeStr=Inherit: Same as first input
  Sum2 : Sum  Inputs=+-  InputSameDT=on  SaturateOnIntegerOverflow=on  OutDataTypeStr=Inherit: Same as first input
  d : UnitDelay  SampleTime=Ts
  d1 : UnitDelay  SampleTime=Ts
  gain : Gain  Gain=2/Ts  SaturateOnIntegerOverflow=on  OutDataTypeStr=Inherit: Same as input  ParamDataTypeStr=Inherit: Same as input
  out : Outport  VectorParamsAs1DForOutWhenUnconnected=off
  wires:
  Sum1/1 -> d1/1, out/1
  d1/1 -> Sum1/2
  Sum2/1 -> gain/1
  in/1 -> d/1, Sum2/1
  d/1 -> Sum2/2
  gain/1 -> Sum1/1

== system Katex_FullCar_R2017b_V03/DGIST/_Low_Level_Ctrl/Steering_Low_Level_Controller/Torque Mode/Steering Motor Control/Feedforward(theta)/Dot1 ==
  note: Dot
  in : Inport
  Sum1 : Sum  Inputs=+-  InputSameDT=on  SaturateOnIntegerOverflow=on  OutDataTypeStr=Inherit: Same as first input
  Sum2 : Sum  Inputs=+-  InputSameDT=on  SaturateOnIntegerOverflow=on  OutDataTypeStr=Inherit: Same as first input
  d : UnitDelay  SampleTime=Ts
  d1 : UnitDelay  SampleTime=Ts
  gain : Gain  Gain=2/Ts  SaturateOnIntegerOverflow=on  OutDataTypeStr=Inherit: Same as input  ParamDataTypeStr=Inherit: Same as input
  out : Outport  VectorParamsAs1DForOutWhenUnconnected=off
  wires:
  Sum1/1 -> d1/1, out/1
  d1/1 -> Sum1/2
  Sum2/1 -> gain/1
  in/1 -> d/1, Sum2/1
  d/1 -> Sum2/2
  gain/1 -> Sum1/1

== system Katex_FullCar_R2017b_V03/DGIST/_Low_Level_Ctrl/Steering_Low_Level_Controller/Torque Mode/Steering Motor Control/Feedforward(theta)/Dot2 ==
  note: Dot
  in : Inport
  Sum1 : Sum  Inputs=+-  InputSameDT=on  SaturateOnIntegerOverflow=on  OutDataTypeStr=Inherit: Same as first input
  Sum2 : Sum  Inputs=+-  InputSameDT=on  SaturateOnIntegerOverflow=on  OutDataTypeStr=Inherit: Same as first input
  d : UnitDelay  SampleTime=Ts
  d1 : UnitDelay  SampleTime=Ts
  gain : Gain  Gain=2/Ts  SaturateOnIntegerOverflow=on  OutDataTypeStr=Inherit: Same as input  ParamDataTypeStr=Inherit: Same as input
  out : Outport  VectorParamsAs1DForOutWhenUnconnected=off
  wires:
  Sum1/1 -> d1/1, out/1
  d1/1 -> Sum1/2
  Sum2/1 -> gain/1
  in/1 -> d/1, Sum2/1
  d/1 -> Sum2/2
  gain/1 -> Sum1/1

== system Katex_FullCar_R2017b_V03/DGIST/_Low_Level_Ctrl/Steering_Low_Level_Controller/Torque Mode/Steering Motor Control/Feedforward(theta)/Second order LPF ==
  note: y(n) = [Ts^2*w^2*{x(n)+2*x(n-1)+x(n-2)}-(2*w^2*Ts^2-8)*y(n-1)-(4+w^2*Ts^2+2*zeta*Ts*w)*y(n-2)]
      | /(4+w^2*Ts^2+2*zeta*Ts*w)
  note: H(s) = w^2/(s^2+2*zeta*w*s+w^2)
  note: s = 2/Ts*(z-1)/(z+1)
  In : Inport
  fc : Inport  Port=2
  zeta : Inport  Port=3
  Constant : Constant  Value=Ts  SampleTime=Ts
  Constant1 : Constant  Value=8  SampleTime=Ts
  Constant2 : Constant  Value=4  SampleTime=Ts
  Delay : Delay  InitialCondition=0  SampleTime=Ts
  Delay1 : Delay  DelayLength=1  InitialCondition=0  SampleTime=Ts
  Delay2 : Delay  DelayLength=1  InitialCondition=0  SampleTime=Ts
  Delay3 : Delay  InitialCondition=0  SampleTime=Ts
  Product1 : Product  Inputs=*/  RndMeth=Zero
  Product2 : Product  Inputs=4  RndMeth=Zero
  Product3 : Product  RndMeth=Zero
  Product4 : Product  RndMeth=Zero
  Sum1 : Sum  Inputs=+-  InputSameDT=on  SaturateOnIntegerOverflow=on  OutDataTypeStr=Inherit: Same as first input
  Sum2 : Sum  Inputs=+-  InputSameDT=on  SaturateOnIntegerOverflow=on  OutDataTypeStr=Inherit: Same as first input
  Sum3 : Sum  Inputs=+++  InputSameDT=on  SaturateOnIntegerOverflow=on  OutDataTypeStr=Inherit: Same as first input
  Sum4 : Sum  Inputs=+-  InputSameDT=on  SaturateOnIntegerOverflow=on  OutDataTypeStr=Inherit: Same as first input
  Sum5 : Sum  Inputs=+-+  InputSameDT=on  SaturateOnIntegerOverflow=on  OutDataTypeStr=Inherit: Same as first input
  Sum6 : Sum  Inputs=+++  InputSameDT=on  SaturateOnIntegerOverflow=on  OutDataTypeStr=Inherit: Same as first input
  gain1 : Gain  Gain=2  SaturateOnIntegerOverflow=on  OutDataTypeStr=Inherit: Same as input  ParamDataTypeStr=Inherit: Same as input
  gain2 : Gain  Gain=2*pi  SaturateOnIntegerOverflow=on  OutDataTypeStr=Inherit: Same as input  ParamDataTypeStr=Inherit: Same as input
  gain3 : Gain  Gain=2  SaturateOnIntegerOverflow=on  OutDataTypeStr=Inherit: Same as input  ParamDataTypeStr=Inherit: Same as input
  gain4 : Gain  Gain=4  SaturateOnIntegerOverflow=on  OutDataTypeStr=Inherit: Same as input  ParamDataTypeStr=Inherit: Same as input
  "x(n), x(n-1), x(n-2)" : Product  RndMeth=Zero
  y(n-1) : Product  RndMeth=Zero
  y(n-2) : Product  RndMeth=Zero
  Out : Outport  VectorParamsAs1DForOutWhenUnconnected=off
  wires:
  Product1/1 -> Out/1, Delay3/1, Delay2/1
  Sum2/1 -> Product1/1
  fc/1 -> gain2/1
  In/1 -> Delay1/1, Delay/1, Sum3/1
  gain2/1 -> Product3/1, Product2/2, Product2/1
  Constant/1 -> Product3/2, Product2/4, Product2/3
  Delay1/1 -> gain1/1
  gain1/1 -> Sum3/2
  Delay/1 -> Sum3/3
  Sum3/1 -> "x(n), x(n-1), x(n-2)"/1
  Product2/1 -> Sum5/1, Sum6/1, "x(n), x(n-1), x(n-2)"/2, gain3/1
  "x(n), x(n-1), x(n-2)"/1 -> Sum1/1
  Sum1/1 -> Sum2/1
  y(n-1)/1 -> Sum1/2
  Sum4/1 -> y(n-1)/1
  gain3/1 -> Sum4/1
  Constant1/1 -> Sum4/2
  Delay2/1 -> y(n-1)/2
  Product3/1 -> gain4/1
  Constant2/1 -> Sum5/3, Sum6/3
  Sum5/1 -> y(n-2)/1
  Delay3/1 -> y(n-2)/2
  y(n-2)/1 -> Sum2/2
  Sum6/1 -> Product1/2
  zeta/1 -> Product4/2
  gain4/1 -> Product4/1
  Product4/1 -> Sum6/2, Sum5/2

== system Katex_FullCar_R2017b_V03/DGIST/_Low_Level_Ctrl/Steering_Low_Level_Controller/Torque Mode/Steering Motor Control/Lag compensator(zeta)/Dot1 ==
  note: Dot
  in : Inport
  Sum1 : Sum  Inputs=+-  InputSameDT=on  SaturateOnIntegerOverflow=on  OutDataTypeStr=Inherit: Same as first input
  Sum2 : Sum  Inputs=+-  InputSameDT=on  SaturateOnIntegerOverflow=on  OutDataTypeStr=Inherit: Same as first input
  d : UnitDelay  SampleTime=Ts
  d1 : UnitDelay  SampleTime=Ts
  gain : Gain  Gain=2/Ts  SaturateOnIntegerOverflow=on  OutDataTypeStr=Inherit: Same as input  ParamDataTypeStr=Inherit: Same as input
  out : Outport  VectorParamsAs1DForOutWhenUnconnected=off
  wires:
  Sum1/1 -> d1/1, out/1
  d1/1 -> Sum1/2
  Sum2/1 -> gain/1
  in/1 -> d/1, Sum2/1
  d/1 -> Sum2/2
  gain/1 -> Sum1/1
